simulink model "aufg1_schaltbild"  (R2015a)
settings: Solver=ode45  StartTime=0.0  StopTime=10.0  RelTol=1e-3
settings Model: Creator=Daniel  LastModifiedBy=Daniel

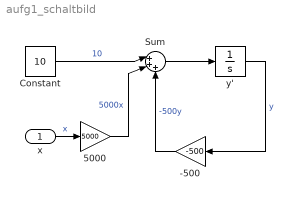
== system aufg1_schaltbild ==
  x : Inport
  -500 : Gain  Gain=-500
  5000 : Gain  Gain=5000
  Constant : Constant  Value=10
  Sum : Sum  Inputs=|+++
  y' : Integrator
  wires:
  Sum/1 -> y'/1
  Constant/1 -> Sum/1  "10"
  y'/1 -> -500/1  "y"
  -500/1 -> Sum/3  "-500y"
  x/1 -> 5000/1  "x"
  5000/1 -> Sum/2  "5000x"
